simulink model "DAS"  (R2012b)
settings: Solver=FixedStepDiscrete  StartTime=0.0  StopTime=inf  FixedStep=0.1  RelTol=1e-3
PreLoadFcn:
  | if exist('tl_preloadfcn','file'), tl_preloadfcn(gcs,101); end
PostLoadFcn:
  | if exist('tl_postloadfcn','file'), tl_postloadfcn(gcs,101); end
InitFcn:
  | if exist('tlds_init','file'), tlds_init(gcs); end
StartFcn:
  | if exist('tlds_start','file'), tlds_start(gcs); end
StopFcn:
  | if exist('tlds_stop','file'), tlds_stop(gcs); end
undefined symbols (not defined in the file): A, B, C, Dd, DEMO_FAS_Accusti_Threshold_Time, DEMO_FAS_BrakeBooster_Threshold, DEMO_FAS_CC_DELTA, DEMO_FAS_CC_Lvl2_Round, DEMO_FAS_CC_Min_Value, DEMO_FAS_Distance_Treshold_Far, DEMO_FAS_Distance_Treshold_Med, DEMO_FAS_Distance_Treshold_Near, DEMO_FAS_Distronic, DEMO_FAS_Emerg_Brake_Force1, DEMO_FAS_Emerg_Brake_Force2, DEMO_FAS_Emerg_Brake_Time1, DEMO_FAS_Emerg_Brake_Time2, DEMO_FAS_EmergencyBrake, DEMO_FAS_FollowToStop, DEMO_FAS_Limiter, DEMO_FAS_Limiter_DELTA, DEMO_FAS_Neg_Max_ms, DEMO_FAS_Opti_Threshold_Time, DEMO_FAS_Repeater, DEMO_FAS_Repeater_Time, DEMO_FAS_Signdetection, DEMO_FAS_Tempomat
(part 3 of 11)

== system DAS/DEMO_FAS/DEMO_FAS/Subsystem/DEMO_FAS/DEMO_FAS_Funktion/EmergencyBrake ==
  V_Vehicle_ms : Inport
  Distance_Object_m : Inport  Port=2
  V_Obj_rel_ms : Inport  Port=3
  DEMO_FAS_EmergencyBrake : Constant  Description=|  Value=DEMO_FAS_EmergencyBrake  SampleTime=-1  mask(TL_Constant){data={'output',{'variable','DEMO_FAS/p/Components/DEMO_FAS_EmergencyBrake'},'date',735389.66817369207}}
      | Constant block of dSPACE TargetLink.
      | 
      | Output signal keeps the given constant value.
      settings: DeleteFcn=if exist('delete_tlblock','file')==2,delete_tlblock(gcbh);end  NameChangeFcn=if exist('rename_tlblock','file')==2,rename_tlblock(gcbh);end  OpenFcn=if exist('tl_open_blockdlg','file')==2,tl_open_blockdlg(gcbh);else,open_system(gcbh,'parameter');end
      mask Help: eval(['if exist(''tl_online_help'',''file'') == 2, tl_online_help(''Topic'',''TL_Constant''),else, web([''jar:file:///'',matlabroot,''/help/toolbox/simulink/help.jar!/slref/' lower(get_param(gcbh,'Blocktype')) '.html''], ''-helpbrowser''),end'])
      mask Display: plot([-0.05, 1.05, NaN, -0.05, 1.05],[.01, .01, NaN, .99, .99])
  EmergencyBrake_Function : Subsystem
  VERSION_INFO : Subsystem  mask(VERSION_INFO_BLOCK){versinfo_data=struct('modname','DEMO_FAS/DEMO_FAS_Funktion/EmergencyBrake','version','1.1.1','date','29-May-2013','author','YVEDUHR','modtype',3,'variant',0,'remark',{{'~'}},'copyright',['Daimler AG'],'SGMLdescr','','prefix','','pfx_act',0,'ntselect',3,'asize',0), versinfo_string=Model: DEMO_FAS/DEMO_FAS_Funktion/EmergencyBrake\nVersion: 1.1.1\nDate: 29-May-2013\nAuthor: YVEDUHR\nModule: INTERNAL\n\nAll copyrights by Daimler AG}
      mask prompts: versinfo_data "Mask Parameter 1"; versinfo_string "Mask Parameter 2"
      mask help:
      | This is a Version Info Subsystem (empty)
      | All version Information is stored in Parameter "versinfo_data" and displayed
      settings: OpenFcn=edit_subsys_info('init')
      mask Display: disp(versinfo_string);
  BrakeForce_Emergency_pc : Outport
  Acusti_warn_b : Outport  Port=2  InitialOutput=0
  wires:
  DEMO_FAS_EmergencyBrake/1 -> EmergencyBrake_Function/Enable
  V_Obj_rel_ms/1 -> EmergencyBrake_Function/3(V_Obj_rel_ms)
  V_Vehicle_ms/1 -> EmergencyBrake_Function/1(V_Vehicle_ms)
  Distance_Object_m/1 -> EmergencyBrake_Function/2(Distance_Object_m)
  EmergencyBrake_Function/1(BrakeForce_Emergency_pc) -> BrakeForce_Emergency_pc/1
  EmergencyBrake_Function/2(Acusti_warn_b) -> Acusti_warn_b/1

== system DAS/DEMO_FAS/DEMO_FAS/Subsystem/DEMO_FAS/DEMO_FAS_Funktion/FAS_Input ==
  InputBus : Inport
  Bus Creator : BusCreator  Inputs=15
  Bus Selector : BusSelector  OutputSignals=ParkingBrake_b,BrakeForce_pedal_pc,Accelaration_pedal_pc,CruiseControl_b,Limiter_b,LeverUp_stat,LeverDown_stat,V_Vehicle_kmh,V_Sign_kmh,Sign_b,Distance_stat,V_Obj_rel_kmh,Distance_Object_m
  Constant : Constant  Value=3.6  mask(TL_Constant){data={'date',735377.63076421292}}
      settings: CopyFcn=if exist('tl_reset_reviewflag') == 2, tl_reset_reviewflag(gcbh); end  DeleteFcn=if exist('delete_tlblock','file')==2,delete_tlblock(gcbh);end  NameChangeFcn=if exist('rename_tlblock','file')==2,rename_tlblock(gcbh);end  OpenFcn=if exist('tl_open_blockdlg','file')==2,tl_open_blockdlg(gcbh);else,open_system(gcbh,'parameter');end
      mask Help: eval(['if exist(''tl_online_help'',''file'') == 2, tl_online_help(''Topic'',''TL_Constant''),else, web([''jar:file:///'',matlabroot,''/help/toolbox/simulink/help.jar!/slref/' lower(get_param(gcbh,'Blocktype')) '.html''], ''-helpbrowser''),end'])
      mask Display: plot([-0.05, 1.05, NaN, -0.05, 1.05],[.01, .01, NaN, .99, .99])
  Constant1 : Constant  Value=3.6  mask(TL_Constant){data={'date',735377.63076421292}}
      settings: CopyFcn=if exist('tl_reset_reviewflag') == 2, tl_reset_reviewflag(gcbh); end  DeleteFcn=if exist('delete_tlblock','file')==2,delete_tlblock(gcbh);end  NameChangeFcn=if exist('rename_tlblock','file')==2,rename_tlblock(gcbh);end  OpenFcn=if exist('tl_open_blockdlg','file')==2,tl_open_blockdlg(gcbh);else,open_system(gcbh,'parameter');end
      mask Help: eval(['if exist(''tl_online_help'',''file'') == 2, tl_online_help(''Topic'',''TL_Constant''),else, web([''jar:file:///'',matlabroot,''/help/toolbox/simulink/help.jar!/slref/' lower(get_param(gcbh,'Blocktype')) '.html''], ''-helpbrowser''),end'])
      mask Display: plot([-0.05, 1.05, NaN, -0.05, 1.05],[.01, .01, NaN, .99, .99])
  Div : Product  Description=|  Inputs=*/  RndMeth=Zero  mask(TL_Product){data={'logdata',{'plotchannels',[]},'date',734383.73388777778}}
      | Product block of dSPACE TargetLink.
      | 
      | Output signal is equal to the product of the input signals. The input ports are specified according to conventions for Simulink Product blocks.
      settings: CopyFcn=if exist('tl_reset_reviewflag') == 2, tl_reset_reviewflag(gcbh); end  DeleteFcn=if exist('delete_tlblock','file')==2,delete_tlblock(gcbh);end  NameChangeFcn=if exist('rename_tlblock','file')==2,rename_tlblock(gcbh);end  OpenFcn=if exist('tl_open_blockdlg','file')==2,tl_open_blockdlg(gcbh);else,open_system(gcbh,'parameter');end
      mask Help: eval(['if exist(''tl_online_help'',''file'') == 2, tl_online_help(''Topic'',''TL_Product''),else, web([''jar:file:///'',matlabroot,''/help/toolbox/simulink/help.jar!/slref/' lower(get_param(gcbh,'Blocktype')) '.html''], ''-helpbrowser''),end'])
      mask Display: plot([-0.05, 1.05, NaN, -0.05, 1.05],[.01, .01, NaN, .99, .99])
  Div1 : Product  Description=|  Inputs=*/  RndMeth=Zero  mask(TL_Product){data={'logdata',{'plotchannels',[]},'date',734383.73388777778}}
      | Product block of dSPACE TargetLink.
      | 
      | Output signal is equal to the product of the input signals. The input ports are specified according to conventions for Simulink Product blocks.
      settings: CopyFcn=if exist('tl_reset_reviewflag') == 2, tl_reset_reviewflag(gcbh); end  DeleteFcn=if exist('delete_tlblock','file')==2,delete_tlblock(gcbh);end  NameChangeFcn=if exist('rename_tlblock','file')==2,rename_tlblock(gcbh);end  OpenFcn=if exist('tl_open_blockdlg','file')==2,tl_open_blockdlg(gcbh);else,open_system(gcbh,'parameter');end
      mask Help: eval(['if exist(''tl_online_help'',''file'') == 2, tl_online_help(''Topic'',''TL_Product''),else, web([''jar:file:///'',matlabroot,''/help/toolbox/simulink/help.jar!/slref/' lower(get_param(gcbh,'Blocktype')) '.html''], ''-helpbrowser''),end'])
      mask Display: plot([-0.05, 1.05, NaN, -0.05, 1.05],[.01, .01, NaN, .99, .99])
  VERSION_INFO : Subsystem  mask(VERSION_INFO_BLOCK){versinfo_data=struct('modname','DEMO_FAS/DEMO_FAS_Funktion/FAS_Input','version','1.1.1','date','18-Apr-2013','author','YVEDUHR','modtype',3,'variant',0,'remark',{{'~'}},'copyright',['Daimler AG'],'SGMLdescr','','prefix','','pfx_act',0,'ntselect',3,'asize',0), versinfo_string=Model: DEMO_FAS/DEMO_FAS_Funktion/FAS_Input\nVersion: 1.1.1\nDate: 18-Apr-2013\nAuthor: YVEDUHR\nModule: INTERNAL\n\nAll copyrights by Daimler AG}
      mask prompts: versinfo_data "Mask Parameter 1"; versinfo_string "Mask Parameter 2"
      mask help:
      | This is a Version Info Subsystem (empty)
      | All version Information is stored in Parameter "versinfo_data" and displayed
      settings: OpenFcn=edit_subsys_info('init')
      mask Display: disp(versinfo_string);
  FASBus : Outport
  wires:
  InputBus/1 -> Bus Selector/1
  Bus Creator/1 -> FASBus/1  "FASBus"
  Bus Selector/1 -> Bus Creator/1  "<ParkingBrake_b>"
  Bus Selector/6 -> Bus Creator/6  "<LeverUp_stat>"
  Bus Selector/4 -> Bus Creator/4  "<CruiseControl_b>"
  Bus Selector/3 -> Bus Creator/3  "<Accelaration_pedal_pc>"
  Bus Selector/2 -> Bus Creator/2  "<BrakeForce_pedal_pc>"
  Bus Selector/8 -> Div/1, Bus Creator/8  "<V_Vehicle_kmh>"
  Bus Selector/5 -> Bus Creator/5  "<Limiter_b>"
  Bus Selector/7 -> Bus Creator/7  "<LeverDown_stat>"
  Bus Selector/9 -> Bus Creator/10  "<V_Sign_kmh>"
  Bus Selector/10 -> Bus Creator/11  "<Sign_b>"
  Bus Selector/13 -> Bus Creator/15  "<Distance_Object_m>"
  Bus Selector/11 -> Bus Creator/12  "<Distance_stat>"
  Constant/1 -> Div/2
  Div/1 -> Bus Creator/9  "V_Vehicle_ms"
  Bus Selector/12 -> Div1/1, Bus Creator/13  "<V_Obj_rel_kmh>"
  Constant1/1 -> Div1/2
  Div1/1 -> Bus Creator/14  "V_Obj_rel_ms"

== system DAS/DEMO_FAS/DEMO_FAS/Subsystem/DEMO_FAS/DEMO_FAS_Funktion/FollowToStop ==
  V_Vehicle_kmh : Inport
  V_Obj_rel_kmh : Inport  Port=2
  DEMO_FAS_FollowToStop : Constant  Description=|  Value=DEMO_FAS_FollowToStop  SampleTime=-1  mask(TL_Constant){data={'output',{'variable','DEMO_FAS/p/Components/DEMO_FAS_Distronic'},'date',735388.55883950228}}
      | Constant block of dSPACE TargetLink.
      | 
      | Output signal keeps the given constant value.
      settings: DeleteFcn=if exist('delete_tlblock','file')==2,delete_tlblock(gcbh);end  NameChangeFcn=if exist('rename_tlblock','file')==2,rename_tlblock(gcbh);end  OpenFcn=if exist('tl_open_blockdlg','file')==2,tl_open_blockdlg(gcbh);else,open_system(gcbh,'parameter');end
      mask Help: eval(['if exist(''tl_online_help'',''file'') == 2, tl_online_help(''Topic'',''TL_Constant''),else, web([''jar:file:///'',matlabroot,''/help/toolbox/simulink/help.jar!/slref/' lower(get_param(gcbh,'Blocktype')) '.html''], ''-helpbrowser''),end'])
      mask Display: plot([-0.05, 1.05, NaN, -0.05, 1.05],[.01, .01, NaN, .99, .99])
  FollowToStop_Function : Subsystem
  VERSION_INFO : Subsystem  mask(VERSION_INFO_BLOCK){versinfo_data=struct('modname','DEMO_FAS/DEMO_FAS_Funktion/FollowToStop','version','1.1.1','date','28-May-2013','author','YVEDUHR','modtype',3,'variant',0,'remark',{{'~'}},'copyright',['Daimler AG'],'SGMLdescr','','prefix','','pfx_act',0,'ntselect',3,'asize',0), versinfo_string=Model: DEMO_FAS/DEMO_FAS_Funktion/FollowToStop\nVersion: 1.1.1\nDate: 28-May-2013\nAuthor: YVEDUHR\nModule: INTERNAL\n\nAll copyrights by Daimler AG}
      mask prompts: versinfo_data "Mask Parameter 1"; versinfo_string "Mask Parameter 2"
      mask help:
      | This is a Version Info Subsystem (empty)
      | All version Information is stored in Parameter "versinfo_data" and displayed
      settings: OpenFcn=edit_subsys_info('init')
      mask Display: disp(versinfo_string);
  FTS_active_b : Outport
  FTS_Abstand_soll_m : Outport  Port=2
  wires:
  V_Vehicle_kmh/1 -> FollowToStop_Function/1(V_Vehicle_kmh)
  V_Obj_rel_kmh/1 -> FollowToStop_Function/2(V_Obj_rel_kmh)
  DEMO_FAS_FollowToStop/1 -> FollowToStop_Function/Enable
  FollowToStop_Function/1(FTS_active_b) -> FTS_active_b/1
  FollowToStop_Function/2(FTS_Abstand_soll_m) -> FTS_Abstand_soll_m/1

== system DAS/DEMO_FAS/DEMO_FAS/Subsystem/DEMO_FAS/DEMO_FAS_Funktion/Limiter ==
  Limiter_b : Inport
  Accelaration_pedal_pc : Inport  Port=2
  V_Vehicle_kmh : Inport  Port=3
  LeverUp_stat : Inport  Port=4
  LeverDown_stat : Inport  Port=5
  V_Sign_kmh : Inport  Port=6
  Sign_b : Inport  Port=7
  DEMO_FAS_Limiter : Constant  Description=|  Value=DEMO_FAS_Limiter  SampleTime=-1  mask(TL_Constant){data={'output',{'variable','DEMO_FAS/p/Components/DEMO_FAS_Limiter'},'date',735342.475759294}}
      | Constant block of dSPACE TargetLink.
      | 
      | Output signal keeps the given constant value.
      settings: DeleteFcn=if exist('delete_tlblock','file')==2,delete_tlblock(gcbh);end  NameChangeFcn=if exist('rename_tlblock','file')==2,rename_tlblock(gcbh);end  OpenFcn=if exist('tl_open_blockdlg','file')==2,tl_open_blockdlg(gcbh);else,open_system(gcbh,'parameter');end
      mask Help: eval(['if exist(''tl_online_help'',''file'') == 2, tl_online_help(''Topic'',''TL_Constant''),else, web([''jar:file:///'',matlabroot,''/help/toolbox/simulink/help.jar!/slref/' lower(get_param(gcbh,'Blocktype')) '.html''], ''-helpbrowser''),end'])
      mask Display: plot([-0.05, 1.05, NaN, -0.05, 1.05],[.01, .01, NaN, .99, .99])
  Limiter_Function : Subsystem
  VERSION_INFO : Subsystem  mask(VERSION_INFO_BLOCK){versinfo_data=struct('modname','DEMO_FAS/DEMO_FAS_Funktion/Limiter','version','1.1.1','date','18-Apr-2013','author','YVEDUHR','modtype',3,'variant',0,'remark',{{['~15-05-2013: Sign Detection added']}},'copyright',['Daimler AG'],'SGMLdescr','','prefix','','pfx_act',0,'ntselect',3,'asize',0), versinfo_string=Model: DEMO_FAS/DEMO_FAS_Funktion/Limiter\nVersion: 1.1.1\nDate: 18-Apr-2013\nAuthor: YVEDUHR\nModule: INTERNAL\n\nAll copyrights by Daimler AG}
      mask prompts: versinfo_data "Mask Parameter 1"; versinfo_string "Mask Parameter 2"
      mask help:
      | This is a Version Info Subsystem (empty)
      | All version Information is stored in Parameter "versinfo_data" and displayed
      settings: OpenFcn=edit_subsys_info('init')
      mask Display: disp(versinfo_string);
  VMax_kmh : Outport
  Limiter_active_b : Outport  Port=2  InitialOutput=0
  wires:
  Limiter_b/1 -> Limiter_Function/1(Limiter_b)
  Accelaration_pedal_pc/1 -> Limiter_Function/2(Accelaration_pedal_pc)
  V_Vehicle_kmh/1 -> Limiter_Function/3(V_Vehicle_kmh)
  LeverUp_stat/1 -> Limiter_Function/4(LeverUp_stat)
  LeverDown_stat/1 -> Limiter_Function/5(LeverDown_stat)
  V_Sign_kmh/1 -> Limiter_Function/6(V_Sign_kmh)
  Sign_b/1 -> Limiter_Function/7(Sign_b)
  Limiter_Function/1(VMax_kmh) -> VMax_kmh/1
  Limiter_Function/2(Limiter_active_b) -> Limiter_active_b/1
  DEMO_FAS_Limiter/1 -> Limiter_Function/Enable

== system DAS/DEMO_FAS/DEMO_FAS/Subsystem/DEMO_FAS/DEMO_FAS_Funktion/Tempomat ==
  ParkingBrake_b : Inport
  BrakeForce_pedal_pc : Inport  Port=2
  CruiseControl_b : Inport  Port=3
  V_Vehicle_kmh : Inport  Port=4
  Limiter_b : Inport  Port=5
  LeverUp_Stat : Inport  Port=6
  LeverDown_Stat : Inport  Port=7
  FTS_active_b : Inport  Port=8
  DEMO_FAS_Tempomat : Constant  Description=|  Value=DEMO_FAS_Tempomat  SampleTime=-1  mask(TL_Constant){data={'output',{'variable','DEMO_FAS/p/Components/DEMO_FAS_Tempomat'},'date',735441.60748548608}}
      | Constant block of dSPACE TargetLink.
      | 
      | Output signal keeps the given constant value.
      settings: DeleteFcn=if exist('delete_tlblock','file')==2,delete_tlblock(gcbh);end  NameChangeFcn=if exist('rename_tlblock','file')==2,rename_tlblock(gcbh);end  OpenFcn=if exist('tl_open_blockdlg','file')==2,tl_open_blockdlg(gcbh);else,open_system(gcbh,'parameter');end
      mask Help: eval(['if exist(''tl_online_help'',''file'') == 2, tl_online_help(''Topic'',''TL_Constant''),else, web([''jar:file:///'',matlabroot,''/help/toolbox/simulink/help.jar!/slref/' lower(get_param(gcbh,'Blocktype')) '.html''], ''-helpbrowser''),end'])
      mask Display: plot([-0.05, 1.05, NaN, -0.05, 1.05],[.01, .01, NaN, .99, .99])
  Tempomat_Function : Subsystem
  VERSION_INFO : Subsystem  mask(VERSION_INFO_BLOCK){versinfo_data=struct('modname','DEMO_FAS/DEMO_FAS_Funktion/Tempomat','version','1.1.1','date','18-Apr-2013','author','YVEDUHR','modtype',3,'variant',0,'remark',{{'~'}},'copyright',['Daimler AG'],'SGMLdescr','','prefix','','pfx_act',0,'ntselect',3,'asize',0), versinfo_string=Model: DEMO_FAS/DEMO_FAS_Funktion/Tempomat\nVersion: 1.1.1\nDate: 18-Apr-2013\nAuthor: YVEDUHR\nModule: INTERNAL\n\nAll copyrights by Daimler AG}
      mask prompts: versinfo_data "Mask Parameter 1"; versinfo_string "Mask Parameter 2"
      mask help:
      | This is a Version Info Subsystem (empty)
      | All version Information is stored in Parameter "versinfo_data" and displayed
      settings: OpenFcn=edit_subsys_info('init')
      mask Display: disp(versinfo_string);
  V_CC_delta_kmh : Outport
  CC_active_b : Outport  Port=2  InitialOutput=0
  wires:
  ParkingBrake_b/1 -> Tempomat_Function/1(ParkingBrake_b)
  BrakeForce_pedal_pc/1 -> Tempomat_Function/2(BrakeForce_pedal_pc)
  CruiseControl_b/1 -> Tempomat_Function/3(CruiseControl_b)
  V_Vehicle_kmh/1 -> Tempomat_Function/4(V_Vehicle_kmh)
  Limiter_b/1 -> Tempomat_Function/5(Limiter_b)
  LeverUp_Stat/1 -> Tempomat_Function/6(LeverUp_Stat)
  LeverDown_Stat/1 -> Tempomat_Function/7(LeverDown_Stat)
  FTS_active_b/1 -> Tempomat_Function/8(FTS_active_b)
  Tempomat_Function/1(V_CC_delta_kmh) -> V_CC_delta_kmh/1
  Tempomat_Function/2(CC_active_b) -> CC_active_b/1
  DEMO_FAS_Tempomat/1 -> Tempomat_Function/Enable

== system DAS/DEMO_FAS/DEMO_FAS/Subsystem/DEMO_FAS/DEMO_FAS_Funktion/VERSION_INFO ==
  Copyright : Subsystem
      mask help: Copyright
      mask Display: disp('All copyrights by DaimlerChrysler');

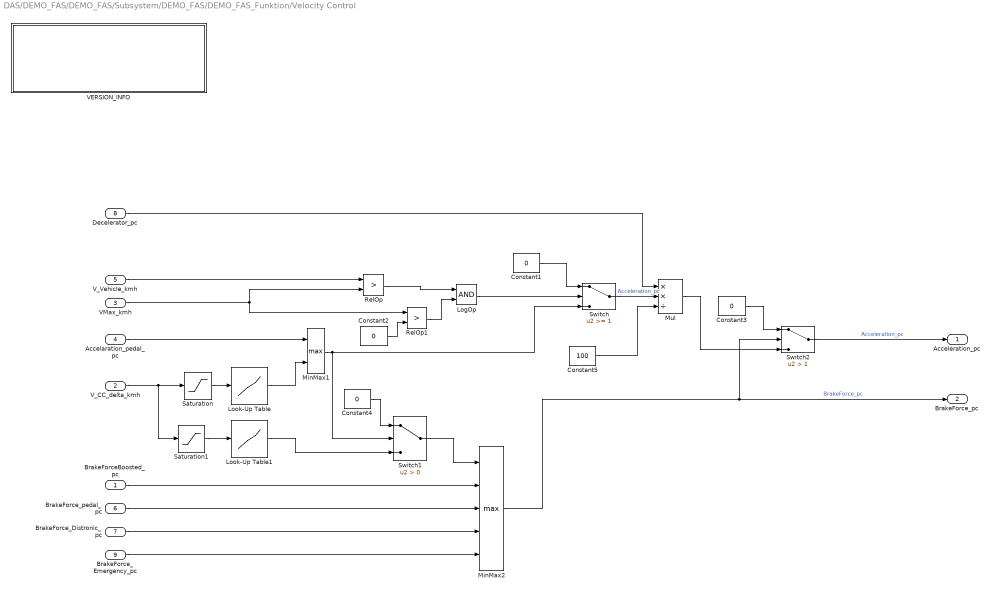
== system DAS/DEMO_FAS/DEMO_FAS/Subsystem/DEMO_FAS/DEMO_FAS_Funktion/Velocity Control ==
  BrakeForceBoosted_pc : Inport
  V_CC_delta_kmh : Inport  Port=2
  VMax_kmh : Inport  Port=3
  Accelaration_pedal_pc : Inport  Port=4
  V_Vehicle_kmh : Inport  Port=5
  BrakeForce_pedal_pc : Inport  Port=6
  BrakeForce_Distronic_pc : Inport  Port=7
  Decelerator_pc : Inport  Port=8
  BrakeForce_Emergency_pc : Inport  Port=9
  Constant{1..4} (4 alike) : Constant  Value=0  mask(TL_Constant){data={'date',735342.59861445602}}
      settings: CopyFcn=if exist('tl_reset_reviewflag') == 2, tl_reset_reviewflag(gcbh); end  DeleteFcn=if exist('delete_tlblock','file')==2,delete_tlblock(gcbh);end  NameChangeFcn=if exist('rename_tlblock','file')==2,rename_tlblock(gcbh);end  OpenFcn=if exist('tl_open_blockdlg','file')==2,tl_open_blockdlg(gcbh);else,open_system(gcbh,'parameter');end
      mask Help: eval(['if exist(''tl_online_help'',''file'') == 2, tl_online_help(''Topic'',''TL_Constant''),else, web([''jar:file:///'',matlabroot,''/help/toolbox/simulink/help.jar!/slref/' lower(get_param(gcbh,'Blocktype')) '.html''], ''-helpbrowser''),end'])
      mask Display: plot([-0.05, 1.05, NaN, -0.05, 1.05],[.01, .01, NaN, .99, .99])
  Constant5 : Constant  Value=100  mask(TL_Constant){data={'date',735389.67880475696}}
      settings: CopyFcn=if exist('tl_reset_reviewflag') == 2, tl_reset_reviewflag(gcbh); end  DeleteFcn=if exist('delete_tlblock','file')==2,delete_tlblock(gcbh);end  NameChangeFcn=if exist('rename_tlblock','file')==2,rename_tlblock(gcbh);end  OpenFcn=if exist('tl_open_blockdlg','file')==2,tl_open_blockdlg(gcbh);else,open_system(gcbh,'parameter');end
      mask Help: eval(['if exist(''tl_online_help'',''file'') == 2, tl_online_help(''Topic'',''TL_Constant''),else, web([''jar:file:///'',matlabroot,''/help/toolbox/simulink/help.jar!/slref/' lower(get_param(gcbh,'Blocktype')) '.html''], ''-helpbrowser''),end'])
      mask Display: plot([-0.05, 1.05, NaN, -0.05, 1.05],[.01, .01, NaN, .99, .99])
  LogOp : Logic  Description=|  AllPortsSameDT=off  mask(TL_LogicalOperator){data={'logdata',{'plotchannels',[]},'date',734383.73388633097}}
      | Logical operator block of dSPACE TargetLink.
      | 
      | The Logical Operator block performs any of these logical operations on its inputs: AND, OR, NAND, NOR, XOR, and NOT. A nonzero input is treated as TRUE (1), a zero input as FALSE (0). The output depends on the selected operator. The output is 1 if TRUE and 0 if FALSE.
      settings: DeleteFcn=if exist('delete_tlblock','file')==2,delete_tlblock(gcbh);end  NameChangeFcn=if exist('rename_tlblock','file')==2,rename_tlblock(gcbh);end  OpenFcn=if exist('tl_open_blockdlg','file')==2,tl_open_blockdlg(gcbh);else,open_system(gcbh,'parameter');end
      mask Help: eval(['if exist(''tl_online_help'',''file'') == 2, tl_online_help(''Topic'',''TL_LogicalOperator''),else, web([''jar:file:///'',matlabroot,''/help/toolbox/simulink/help.jar!/slref/' lower(get_param(gcbh,'Blocktype')) '.html''], ''-helpbrowser''),end'])
      mask Display: plot([-0.05, 1.05, NaN, -0.05, 1.05],[.01, .01, NaN, .99, .99])
  Look-Up Table : Lookup_n-D  NumberOfTableDimensions=1  BreakpointsForDimension1=[0 1 5 10]  BreakpointsForDimension2=[1:3]  IndexSearchMethod=Linear search  Table=[0 20 60 100]  ExtrapMethod=Clip  RndMeth=Simplest  InputSameDT=on  mask(TL_Lookup1D){data={'input',{'type','Int16'},'table',{'type','Int16'},'date',735342.59760248847}}
      settings: CopyFcn=if exist('tl_reset_reviewflag') == 2, tl_reset_reviewflag(gcbh); end  DeleteFcn=if exist('delete_tlblock','file')==2,delete_tlblock(gcbh);end  NameChangeFcn=if exist('rename_tlblock','file')==2,rename_tlblock(gcbh);end  OpenFcn=if exist('tl_open_blockdlg','file')==2,tl_open_blockdlg(gcbh);else,open_system(gcbh,'parameter');end
      mask Help: eval(['if exist(''tl_online_help'',''file'') == 2, tl_online_help(''Topic'',''TL_Lookup1D''),else, web([''jar:file:///'',matlabroot,''/help/toolbox/simulink/help.jar!/slref/' lower(get_param(gcbh,'Blocktype')) '.html''], ''-helpbrowser''),end'])
      mask Display: plot([-0.05, 1.05, NaN, -0.05, 1.05],[.01, .01, NaN, .99, .99])
  Look-Up Table1 : Lookup_n-D  NumberOfTableDimensions=1  BreakpointsForDimension1=[-10 -5 -1 0]  BreakpointsForDimension2=[1:3]  IndexSearchMethod=Linear search  Table=[100 40 5 0]  ExtrapMethod=Clip  RndMeth=Simplest  InputSameDT=on  mask(TL_Lookup1D){data={'input',{'type','Int16'},'table',{'type','Int16'},'date',735350.38531726855}}
      settings: CopyFcn=if exist('tl_reset_reviewflag') == 2, tl_reset_reviewflag(gcbh); end  DeleteFcn=if exist('delete_tlblock','file')==2,delete_tlblock(gcbh);end  NameChangeFcn=if exist('rename_tlblock','file')==2,rename_tlblock(gcbh);end  OpenFcn=if exist('tl_open_blockdlg','file')==2,tl_open_blockdlg(gcbh);else,open_system(gcbh,'parameter');end
      mask Help: eval(['if exist(''tl_online_help'',''file'') == 2, tl_online_help(''Topic'',''TL_Lookup1D''),else, web([''jar:file:///'',matlabroot,''/help/toolbox/simulink/help.jar!/slref/' lower(get_param(gcbh,'Blocktype')) '.html''], ''-helpbrowser''),end'])
      mask Display: plot([-0.05, 1.05, NaN, -0.05, 1.05],[.01, .01, NaN, .99, .99])
  MinMax1 : MinMax  Description=|  Function=max  Inputs=2  mask(TL_MinMax){data={'logdata',{'plotchannels',[]},'date',735342.59806893521}}
      | MinMax block of dSPACE TargetLink.
      | 
      | The MinMax block outputs either the minimum or the maximum element or elements of the input(s). If the block has one input port, the block outputs a scalar that is the minimum or maximum element of the input vector. If the block has more than one input port, the block performs an element-by-element comparison of the input vectors. Each element of the block output vector is the result of the comparison of the elements of the input vectors. The output of this block is equal to the greater or smaller input depending on the selected function.
      settings: CopyFcn=if exist('tl_reset_reviewflag') == 2, tl_reset_reviewflag(gcbh); end  DeleteFcn=if exist('delete_tlblock','file')==2,delete_tlblock(gcbh);end  NameChangeFcn=if exist('rename_tlblock','file')==2,rename_tlblock(gcbh);end  OpenFcn=if exist('tl_open_blockdlg','file')==2,tl_open_blockdlg(gcbh);else,open_system(gcbh,'parameter');end
      mask Help: eval(['if exist(''tl_online_help'',''file'') == 2, tl_online_help(''Topic'',''TL_MinMax''),else, web([''jar:file:///'',matlabroot,''/help/toolbox/simulink/help.jar!/slref/' lower(get_param(gcbh,'Blocktype')) '.html''], ''-helpbrowser''),end'])
      mask Display: plot([-0.05, 1.05, NaN, -0.05, 1.05],[.01, .01, NaN, .99, .99])
  MinMax2 : MinMax  Description=|  Function=max  Inputs=5  mask(TL_MinMax){data={'logdata',{'plotchannels',[]},'date',735383.5334921875}}
      | MinMax block of dSPACE TargetLink.
      | 
      | The MinMax block outputs either the minimum or the maximum element or elements of the input(s). If the block has one input port, the block outputs a scalar that is the minimum or maximum element of the input vector. If the block has more than one input port, the block performs an element-by-element comparison of the input vectors. Each element of the block output vector is the result of the comparison of the elements of the input vectors. The output of this block is equal to the greater or smaller input depending on the selected function.
      settings: CopyFcn=if exist('tl_reset_reviewflag') == 2, tl_reset_reviewflag(gcbh); end  DeleteFcn=if exist('delete_tlblock','file')==2,delete_tlblock(gcbh);end  NameChangeFcn=if exist('rename_tlblock','file')==2,rename_tlblock(gcbh);end  OpenFcn=if exist('tl_open_blockdlg','file')==2,tl_open_blockdlg(gcbh);else,open_system(gcbh,'parameter');end
      mask Help: eval(['if exist(''tl_online_help'',''file'') == 2, tl_online_help(''Topic'',''TL_MinMax''),else, web([''jar:file:///'',matlabroot,''/help/toolbox/simulink/help.jar!/slref/' lower(get_param(gcbh,'Blocktype')) '.html''], ''-helpbrowser''),end'])
      mask Display: plot([-0.05, 1.05, NaN, -0.05, 1.05],[.01, .01, NaN, .99, .99])
  Mul : Product  Description=|  Inputs=**/  RndMeth=Zero  mask(TL_Product){data={'logdata',{'plotchannels',[]},'date',735389.67847318284}}
      | Product block of dSPACE TargetLink.
      | 
      | Output signal is equal to the product of the input signals. The input ports are specified according to conventions for Simulink Product blocks.
      settings: CopyFcn=if exist('tl_reset_reviewflag') == 2, tl_reset_reviewflag(gcbh); end  DeleteFcn=if exist('delete_tlblock','file')==2,delete_tlblock(gcbh);end  NameChangeFcn=if exist('rename_tlblock','file')==2,rename_tlblock(gcbh);end  OpenFcn=if exist('tl_open_blockdlg','file')==2,tl_open_blockdlg(gcbh);else,open_system(gcbh,'parameter');end
      mask Help: eval(['if exist(''tl_online_help'',''file'') == 2, tl_online_help(''Topic'',''TL_Product''),else, web([''jar:file:///'',matlabroot,''/help/toolbox/simulink/help.jar!/slref/' lower(get_param(gcbh,'Blocktype')) '.html''], ''-helpbrowser''),end'])
      mask Display: plot([-0.05, 1.05, NaN, -0.05, 1.05],[.01, .01, NaN, .99, .99])
  RelOp : RelationalOperator  Description=|  Operator=>  mask(TL_RelationalOperator){data={'logdata',{'plotchannels',[]},'date',735342.59901829856}}
      | Relational operator block of dSPACE TargetLink.
      | 
      | This block performs a relational operation on its two inputs u1 and u2 and produces output according to the following table.
      | If the result is TRUE, the output is 1; if FALSE, it is 0.
      | 
      | Operator   Output
      |  ==        TRUE if u1 is equal to u2
      |  !=        TRUE if u1 is not equal to u2
      |  <         TRUE if u1 is less than u2
      |  <=        TRUE if u1 is less than or equal to u2
      |  >=        TRUE if u1 is greater than or equal to u2
      |  >         TRUE if u1 is greater than u2
      settings: DeleteFcn=if exist('delete_tlblock','file')==2,delete_tlblock(gcbh);end  NameChangeFcn=if exist('rename_tlblock','file')==2,rename_tlblock(gcbh);end  OpenFcn=if exist('tl_open_blockdlg','file')==2,tl_open_blockdlg(gcbh);else,open_system(gcbh,'parameter');end
      mask Help: eval(['if exist(''tl_online_help'',''file'') == 2, tl_online_help(''Topic'',''TL_RelationalOperator''),else, web([''jar:file:///'',matlabroot,''/help/toolbox/simulink/help.jar!/slref/' lower(get_param(gcbh,'Blocktype')) '.html''], ''-helpbrowser''),end'])
      mask Display: plot([-0.05, 1.05, NaN, -0.05, 1.05],[.01, .01, NaN, .99, .99])
  RelOp1 : RelationalOperator  Description=|  Operator=>  mask(TL_RelationalOperator){data={'logdata',{'plotchannels',[]},'date',735342.59901829856}}
      | Relational operator block of dSPACE TargetLink.
      | 
      | This block performs a relational operation on its two inputs u1 and u2 and produces output according to the following table.
      | If the result is TRUE, the output is 1; if FALSE, it is 0.
      | 
      | Operator   Output
      |  ==        TRUE if u1 is equal to u2
      |  !=        TRUE if u1 is not equal to u2
      |  <         TRUE if u1 is less than u2
      |  <=        TRUE if u1 is less than or equal to u2
      |  >=        TRUE if u1 is greater than or equal to u2
      |  >         TRUE if u1 is greater than u2
      settings: DeleteFcn=if exist('delete_tlblock','file')==2,delete_tlblock(gcbh);end  NameChangeFcn=if exist('rename_tlblock','file')==2,rename_tlblock(gcbh);end  OpenFcn=if exist('tl_open_blockdlg','file')==2,tl_open_blockdlg(gcbh);else,open_system(gcbh,'parameter');end
      mask Help: eval(['if exist(''tl_online_help'',''file'') == 2, tl_online_help(''Topic'',''TL_RelationalOperator''),else, web([''jar:file:///'',matlabroot,''/help/toolbox/simulink/help.jar!/slref/' lower(get_param(gcbh,'Blocktype')) '.html''], ''-helpbrowser''),end'])
      mask Display: plot([-0.05, 1.05, NaN, -0.05, 1.05],[.01, .01, NaN, .99, .99])
  Saturation : Saturate  UpperLimit=10  LowerLimit=0  mask(TL_Saturate){data={'date',735342.62833549769}}
      settings: CopyFcn=if exist('tl_reset_reviewflag') == 2, tl_reset_reviewflag(gcbh); end  DeleteFcn=if exist('delete_tlblock','file')==2,delete_tlblock(gcbh);end  NameChangeFcn=if exist('rename_tlblock','file')==2,rename_tlblock(gcbh);end  OpenFcn=if exist('tl_open_blockdlg','file')==2,tl_open_blockdlg(gcbh);else,open_system(gcbh,'parameter');end
      mask Help: eval(['if exist(''tl_online_help'',''file'') == 2, tl_online_help(''Topic'',''TL_Saturate''),else, web([''jar:file:///'',matlabroot,''/help/toolbox/simulink/help.jar!/slref/' lower(get_param(gcbh,'Blocktype')) '.html''], ''-helpbrowser''),end'])
      mask Display: plot([-0.05, 1.05, NaN, -0.05, 1.05],[.01, .01, NaN, .99, .99])
  Saturation1 : Saturate  UpperLimit=0  LowerLimit=-10  mask(TL_Saturate){data={'date',735350.38457865745}}
      settings: CopyFcn=if exist('tl_reset_reviewflag') == 2, tl_reset_reviewflag(gcbh); end  DeleteFcn=if exist('delete_tlblock','file')==2,delete_tlblock(gcbh);end  NameChangeFcn=if exist('rename_tlblock','file')==2,rename_tlblock(gcbh);end  OpenFcn=if exist('tl_open_blockdlg','file')==2,tl_open_blockdlg(gcbh);else,open_system(gcbh,'parameter');end
      mask Help: eval(['if exist(''tl_online_help'',''file'') == 2, tl_online_help(''Topic'',''TL_Saturate''),else, web([''jar:file:///'',matlabroot,''/help/toolbox/simulink/help.jar!/slref/' lower(get_param(gcbh,'Blocktype')) '.html''], ''-helpbrowser''),end'])
      mask Display: plot([-0.05, 1.05, NaN, -0.05, 1.05],[.01, .01, NaN, .99, .99])
  Switch : Switch  Threshold=1  mask(TL_Switch){data={'date',735342.59663996531}}
      settings: CopyFcn=if exist('tl_reset_reviewflag') == 2, tl_reset_reviewflag(gcbh); end  DeleteFcn=if exist('delete_tlblock','file')==2,delete_tlblock(gcbh);end  NameChangeFcn=if exist('rename_tlblock','file')==2,rename_tlblock(gcbh);end  OpenFcn=if exist('tl_open_blockdlg','file')==2,tl_open_blockdlg(gcbh);else,open_system(gcbh,'parameter');end
      mask Help: eval(['if exist(''tl_online_help'',''file'') == 2, tl_online_help(''Topic'',''TL_Switch''),else, web([''jar:file:///'',matlabroot,''/help/toolbox/simulink/help.jar!/slref/' lower(get_param(gcbh,'Blocktype')) '.html''], ''-helpbrowser''),end'])
      mask Display: plot([-0.05, 1.05, NaN, -0.05, 1.05],[.01, .01, NaN, .99, .99])
  Switch1 : Switch  Criteria=u2 > Threshold  mask(TL_Switch){data={'date',735350.47172620369}}
      settings: CopyFcn=if exist('tl_reset_reviewflag') == 2, tl_reset_reviewflag(gcbh); end  DeleteFcn=if exist('delete_tlblock','file')==2,delete_tlblock(gcbh);end  NameChangeFcn=if exist('rename_tlblock','file')==2,rename_tlblock(gcbh);end  OpenFcn=if exist('tl_open_blockdlg','file')==2,tl_open_blockdlg(gcbh);else,open_system(gcbh,'parameter');end
      mask Help: eval(['if exist(''tl_online_help'',''file'') == 2, tl_online_help(''Topic'',''TL_Switch''),else, web([''jar:file:///'',matlabroot,''/help/toolbox/simulink/help.jar!/slref/' lower(get_param(gcbh,'Blocktype')) '.html''], ''-helpbrowser''),end'])
      mask Display: plot([-0.05, 1.05, NaN, -0.05, 1.05],[.01, .01, NaN, .99, .99])
  Switch2 : Switch  Criteria=u2 > Threshold  Threshold=1  mask(TL_Switch){data={'date',735389.69151828706}}
      settings: CopyFcn=if exist('tl_reset_reviewflag') == 2, tl_reset_reviewflag(gcbh); end  DeleteFcn=if exist('delete_tlblock','file')==2,delete_tlblock(gcbh);end  NameChangeFcn=if exist('rename_tlblock','file')==2,rename_tlblock(gcbh);end  OpenFcn=if exist('tl_open_blockdlg','file')==2,tl_open_blockdlg(gcbh);else,open_system(gcbh,'parameter');end
      mask Help: eval(['if exist(''tl_online_help'',''file'') == 2, tl_online_help(''Topic'',''TL_Switch''),else, web([''jar:file:///'',matlabroot,''/help/toolbox/simulink/help.jar!/slref/' lower(get_param(gcbh,'Blocktype')) '.html''], ''-helpbrowser''),end'])
      mask Display: plot([-0.05, 1.05, NaN, -0.05, 1.05],[.01, .01, NaN, .99, .99])
  VERSION_INFO : Subsystem  mask(VERSION_INFO_BLOCK){versinfo_data=struct('modname',['DEMO_FAS/DEMO_FAS_Funktion/Velocity Control'],'version','1.1.1','date','18-Apr-2013','author','YVEDUHR','modtype',3,'variant',0,'remark',{{'~'}},'copyright',['Daimler AG'],'SGMLdescr','','prefix','','pfx_act',0,'ntselect',3,'asize',0), versinfo_string=Model: DEMO_FAS/DEMO_FAS_Funktion/Velocity Control\nVersion: 1.1.1\nDate: 18-Apr-2013\nAuthor: YVEDUHR\nModule: INTERNAL\n\nAll copyrights by Daimler AG}
      mask prompts: versinfo_data "Mask Parameter 1"; versinfo_string "Mask Parameter 2"
      mask help:
      | This is a Version Info Subsystem (empty)
      | All version Information is stored in Parameter "versinfo_data" and displayed
      settings: OpenFcn=edit_subsys_info('init')
      mask Display: disp(versinfo_string);
  Acceleration_pc : Outport
  BrakeForce_pc : Outport  Port=2
  wires:
  Constant1/1 -> Switch/1
  RelOp1/1 -> LogOp/2
  RelOp/1 -> LogOp/1
  LogOp/1 -> Switch/2
  V_CC_delta_kmh/1 -> Saturation1/1, Saturation/1
  Look-Up Table/1 -> MinMax1/2
  V_Vehicle_kmh/1 -> RelOp/1
  VMax_kmh/1 -> RelOp1/1, RelOp/2
  Accelaration_pedal_pc/1 -> MinMax1/1
  Switch2/1 -> Acceleration_pc/1  "Acceleration_pc"
  Constant2/1 -> RelOp1/2
  Saturation/1 -> Look-Up Table/1
  Saturation1/1 -> Look-Up Table1/1
  BrakeForceBoosted_pc/1 -> MinMax2/2
  Look-Up Table1/1 -> Switch1/3
  BrakeForce_pedal_pc/1 -> MinMax2/3
  MinMax2/1 -> Switch2/2, BrakeForce_pc/1  "BrakeForce_pc"
  Switch1/1 -> MinMax2/1
  MinMax1/1 -> Switch1/2, Switch/3
  Constant4/1 -> Switch1/1
  BrakeForce_Emergency_pc/1 -> MinMax2/5
  BrakeForce_Distronic_pc/1 -> MinMax2/4
  Switch/1 -> Mul/2  "Acceleration_pc"
  Constant3/1 -> Switch2/1
  Decelerator_pc/1 -> Mul/1
  Mul/1 -> Switch2/3
  Constant5/1 -> Mul/3

== system DAS/DEMO_FAS/DEMO_FAS/Subsystem/DEMO_FAS/DEMO_FAS_Funktion/BrakeAssistant/Brake_Booster ==
  BrakeForce_pedal_pc : Inport
  Constant : Constant  Value=100  mask(TL_Constant){data={'date',735349.62176872685}}
      settings: CopyFcn=if exist('tl_reset_reviewflag') == 2, tl_reset_reviewflag(gcbh); end  DeleteFcn=if exist('delete_tlblock','file')==2,delete_tlblock(gcbh);end  NameChangeFcn=if exist('rename_tlblock','file')==2,rename_tlblock(gcbh);end  OpenFcn=if exist('tl_open_blockdlg','file')==2,tl_open_blockdlg(gcbh);else,open_system(gcbh,'parameter');end
      mask Help: eval(['if exist(''tl_online_help'',''file'') == 2, tl_online_help(''Topic'',''TL_Constant''),else, web([''jar:file:///'',matlabroot,''/help/toolbox/simulink/help.jar!/slref/' lower(get_param(gcbh,'Blocktype')) '.html''], ''-helpbrowser''),end'])
      mask Display: plot([-0.05, 1.05, NaN, -0.05, 1.05],[.01, .01, NaN, .99, .99])
  DEMO_FAS_BrakeBooster_Threshold : Constant  Description=|  Value=DEMO_FAS_BrakeBooster_Threshold  SampleTime=-1  mask(TL_Constant){data={'output',{'variable','DEMO_FAS/p/Components/DEMO_FAS_BrakeBooster_Threshold'},'date',735354.40793805558}}
      | Constant block of dSPACE TargetLink.
      | 
      | Output signal keeps the given constant value.
      settings: DeleteFcn=if exist('delete_tlblock','file')==2,delete_tlblock(gcbh);end  NameChangeFcn=if exist('rename_tlblock','file')==2,rename_tlblock(gcbh);end  OpenFcn=if exist('tl_open_blockdlg','file')==2,tl_open_blockdlg(gcbh);else,open_system(gcbh,'parameter');end
      mask Help: eval(['if exist(''tl_online_help'',''file'') == 2, tl_online_help(''Topic'',''TL_Constant''),else, web([''jar:file:///'',matlabroot,''/help/toolbox/simulink/help.jar!/slref/' lower(get_param(gcbh,'Blocktype')) '.html''], ''-helpbrowser''),end'])
      mask Display: plot([-0.05, 1.05, NaN, -0.05, 1.05],[.01, .01, NaN, .99, .99])
  RelOp : RelationalOperator  Description=|  mask(TL_RelationalOperator){data={'logdata',{'plotchannels',[]},'date',735349.6188950463}}
      | Relational operator block of dSPACE TargetLink.
      | 
      | This block performs a relational operation on its two inputs u1 and u2 and produces output according to the following table.
      | If the result is TRUE, the output is 1; if FALSE, it is 0.
      | 
      | Operator   Output
      |  ==        TRUE if u1 is equal to u2
      |  !=        TRUE if u1 is not equal to u2
      |  <         TRUE if u1 is less than u2
      |  <=        TRUE if u1 is less than or equal to u2
      |  >=        TRUE if u1 is greater than or equal to u2
      |  >         TRUE if u1 is greater than u2
      settings: DeleteFcn=if exist('delete_tlblock','file')==2,delete_tlblock(gcbh);end  NameChangeFcn=if exist('rename_tlblock','file')==2,rename_tlblock(gcbh);end  OpenFcn=if exist('tl_open_blockdlg','file')==2,tl_open_blockdlg(gcbh);else,open_system(gcbh,'parameter');end
      mask Help: eval(['if exist(''tl_online_help'',''file'') == 2, tl_online_help(''Topic'',''TL_RelationalOperator''),else, web([''jar:file:///'',matlabroot,''/help/toolbox/simulink/help.jar!/slref/' lower(get_param(gcbh,'Blocktype')) '.html''], ''-helpbrowser''),end'])
      mask Display: plot([-0.05, 1.05, NaN, -0.05, 1.05],[.01, .01, NaN, .99, .99])
  Switch : Switch  Threshold=1  mask(TL_Switch){data={'date',735349.62130812497}}
      settings: CopyFcn=if exist('tl_reset_reviewflag') == 2, tl_reset_reviewflag(gcbh); end  DeleteFcn=if exist('delete_tlblock','file')==2,delete_tlblock(gcbh);end  NameChangeFcn=if exist('rename_tlblock','file')==2,rename_tlblock(gcbh);end  OpenFcn=if exist('tl_open_blockdlg','file')==2,tl_open_blockdlg(gcbh);else,open_system(gcbh,'parameter');end
      mask Help: eval(['if exist(''tl_online_help'',''file'') == 2, tl_online_help(''Topic'',''TL_Switch''),else, web([''jar:file:///'',matlabroot,''/help/toolbox/simulink/help.jar!/slref/' lower(get_param(gcbh,'Blocktype')) '.html''], ''-helpbrowser''),end'])
      mask Display: plot([-0.05, 1.05, NaN, -0.05, 1.05],[.01, .01, NaN, .99, .99])
  VERSION_INFO : Subsystem  mask(VERSION_INFO_BLOCK){versinfo_data=struct('modname','DEMO_FAS/DEMO_FAS_Funktion/BrakeAssistant/Brake_Booster','version','1.1.1','date','26-Apr-2013','author','YVEDUHR','modtype',3,'variant',0,'remark',{{'~'}},'copyright',['Daimler AG'],'SGMLdescr','','prefix','','pfx_act',0,'ntselect',3,'asize',0), versinfo_string=Model: DEMO_FAS/DEMO_FAS_Funktion/BrakeAssistant/Brake_Booster\nVersion: 1.1.1\nDate: 26-Apr-2013\nAuthor: YVEDUHR\nModule: INTERNAL\n\nAll copyrights by Daimler AG}
      mask prompts: versinfo_data "Mask Parameter 1"; versinfo_string "Mask Parameter 2"
      mask help:
      | This is a Version Info Subsystem (empty)
      | All version Information is stored in Parameter "versinfo_data" and displayed
      settings: OpenFcn=edit_subsys_info('init')
      mask Display: disp(versinfo_string);
  BrakeForceBoosted_pc : Outport  OutputWhenDisabled=reset  InitialOutput=0
  wires:
  BrakeForce_pedal_pc/1 -> Switch/3, RelOp/1
  RelOp/1 -> Switch/2
  DEMO_FAS_BrakeBooster_Threshold/1 -> RelOp/2
  Constant/1 -> Switch/1
  Switch/1 -> BrakeForceBoosted_pc/1  "BrakeForceBoosted_pc"

== system DAS/DEMO_FAS/DEMO_FAS/Subsystem/DEMO_FAS/DEMO_FAS_Funktion/BrakeAssistant/VERSION_INFO ==
  Copyright : Subsystem
      mask help: Copyright
      mask Display: disp('All copyrights by DaimlerChrysler');

== system DAS/DEMO_FAS/DEMO_FAS/Subsystem/DEMO_FAS/DEMO_FAS_Funktion/Distancewarner/Distancewarner_Function ==
  V_Vehicle_ms : Inport
  Distance_Object_m : Inport  Port=2
  DEMO_FAS_Accusti_Threshold_Time : Constant  Description=|  Value=DEMO_FAS_Accusti_Threshold_Time  SampleTime=-1  mask(TL_Constant){data={'output',{'variable','DEMO_FAS/p/Components/DEMO_FAS_Accusti_Threshold_Time'},'date',735382.58424127311}}
      | Constant block of dSPACE TargetLink.
      | 
      | Output signal keeps the given constant value.
      settings: DeleteFcn=if exist('delete_tlblock','file')==2,delete_tlblock(gcbh);end  NameChangeFcn=if exist('rename_tlblock','file')==2,rename_tlblock(gcbh);end  OpenFcn=if exist('tl_open_blockdlg','file')==2,tl_open_blockdlg(gcbh);else,open_system(gcbh,'parameter');end
      mask Help: eval(['if exist(''tl_online_help'',''file'') == 2, tl_online_help(''Topic'',''TL_Constant''),else, web([''jar:file:///'',matlabroot,''/help/toolbox/simulink/help.jar!/slref/' lower(get_param(gcbh,'Blocktype')) '.html''], ''-helpbrowser''),end'])
      mask Display: plot([-0.05, 1.05, NaN, -0.05, 1.05],[.01, .01, NaN, .99, .99])
  DEMO_FAS_Opti_Threshold_Time : Constant  Description=|  Value=DEMO_FAS_Opti_Threshold_Time  SampleTime=-1  mask(TL_Constant){data={'output',{'variable','DEMO_FAS/p/Components/DEMO_FAS_Opti_Threshold_Time'},'date',735382.58416377311}}
      | Constant block of dSPACE TargetLink.
      | 
      | Output signal keeps the given constant value.
      settings: DeleteFcn=if exist('delete_tlblock','file')==2,delete_tlblock(gcbh);end  NameChangeFcn=if exist('rename_tlblock','file')==2,rename_tlblock(gcbh);end  OpenFcn=if exist('tl_open_blockdlg','file')==2,tl_open_blockdlg(gcbh);else,open_system(gcbh,'parameter');end
      mask Help: eval(['if exist(''tl_online_help'',''file'') == 2, tl_online_help(''Topic'',''TL_Constant''),else, web([''jar:file:///'',matlabroot,''/help/toolbox/simulink/help.jar!/slref/' lower(get_param(gcbh,'Blocktype')) '.html''], ''-helpbrowser''),end'])
      mask Display: plot([-0.05, 1.05, NaN, -0.05, 1.05],[.01, .01, NaN, .99, .99])
  Mul : Product  Description=|  Inputs=**  RndMeth=Zero  mask(TL_Product){data={'logdata',{'plotchannels',[]},'date',734383.73388434027}}
      | Product block of dSPACE TargetLink.
      | 
      | Output signal is equal to the product of the input signals. The input ports are specified according to conventions for Simulink Product blocks.
      settings: CopyFcn=if exist('tl_reset_reviewflag') == 2, tl_reset_reviewflag(gcbh); end  DeleteFcn=if exist('delete_tlblock','file')==2,delete_tlblock(gcbh);end  NameChangeFcn=if exist('rename_tlblock','file')==2,rename_tlblock(gcbh);end  OpenFcn=if exist('tl_open_blockdlg','file')==2,tl_open_blockdlg(gcbh);else,open_system(gcbh,'parameter');end
      mask Help: eval(['if exist(''tl_online_help'',''file'') == 2, tl_online_help(''Topic'',''TL_Product''),else, web([''jar:file:///'',matlabroot,''/help/toolbox/simulink/help.jar!/slref/' lower(get_param(gcbh,'Blocktype')) '.html''], ''-helpbrowser''),end'])
      mask Display: plot([-0.05, 1.05, NaN, -0.05, 1.05],[.01, .01, NaN, .99, .99])
  Mul1 : Product  Description=|  Inputs=**  RndMeth=Zero  mask(TL_Product){data={'logdata',{'plotchannels',[]},'date',734383.73388434027}}
      | Product block of dSPACE TargetLink.
      | 
      | Output signal is equal to the product of the input signals. The input ports are specified according to conventions for Simulink Product blocks.
      settings: CopyFcn=if exist('tl_reset_reviewflag') == 2, tl_reset_reviewflag(gcbh); end  DeleteFcn=if exist('delete_tlblock','file')==2,delete_tlblock(gcbh);end  NameChangeFcn=if exist('rename_tlblock','file')==2,rename_tlblock(gcbh);end  OpenFcn=if exist('tl_open_blockdlg','file')==2,tl_open_blockdlg(gcbh);else,open_system(gcbh,'parameter');end
      mask Help: eval(['if exist(''tl_online_help'',''file'') == 2, tl_online_help(''Topic'',''TL_Product''),else, web([''jar:file:///'',matlabroot,''/help/toolbox/simulink/help.jar!/slref/' lower(get_param(gcbh,'Blocktype')) '.html''], ''-helpbrowser''),end'])
      mask Display: plot([-0.05, 1.05, NaN, -0.05, 1.05],[.01, .01, NaN, .99, .99])
  RelOp : RelationalOperator  Description=|  Operator=<=  mask(TL_RelationalOperator){data={'logdata',{'plotchannels',[]},'date',734383.73388379626}}
      | Relational operator block of dSPACE TargetLink.
      | 
      | This block performs a relational operation on its two inputs u1 and u2 and produces output according to the following table.
      | If the result is TRUE, the output is 1; if FALSE, it is 0.
      | 
      | Operator   Output
      |  ==        TRUE if u1 is equal to u2
      |  !=        TRUE if u1 is not equal to u2
      |  <         TRUE if u1 is less than u2
      |  <=        TRUE if u1 is less than or equal to u2
      |  >=        TRUE if u1 is greater than or equal to u2
      |  >         TRUE if u1 is greater than u2
      settings: DeleteFcn=if exist('delete_tlblock','file')==2,delete_tlblock(gcbh);end  NameChangeFcn=if exist('rename_tlblock','file')==2,rename_tlblock(gcbh);end  OpenFcn=if exist('tl_open_blockdlg','file')==2,tl_open_blockdlg(gcbh);else,open_system(gcbh,'parameter');end
      mask Help: eval(['if exist(''tl_online_help'',''file'') == 2, tl_online_help(''Topic'',''TL_RelationalOperator''),else, web([''jar:file:///'',matlabroot,''/help/toolbox/simulink/help.jar!/slref/' lower(get_param(gcbh,'Blocktype')) '.html''], ''-helpbrowser''),end'])
      mask Display: plot([-0.05, 1.05, NaN, -0.05, 1.05],[.01, .01, NaN, .99, .99])
  RelOp2 : RelationalOperator  Description=|  Operator=<=  mask(TL_RelationalOperator){data={'logdata',{'plotchannels',[]},'date',734383.73388379626}}
      | Relational operator block of dSPACE TargetLink.
      | 
      | This block performs a relational operation on its two inputs u1 and u2 and produces output according to the following table.
      | If the result is TRUE, the output is 1; if FALSE, it is 0.
      | 
      | Operator   Output
      |  ==        TRUE if u1 is equal to u2
      |  !=        TRUE if u1 is not equal to u2
      |  <         TRUE if u1 is less than u2
      |  <=        TRUE if u1 is less than or equal to u2
      |  >=        TRUE if u1 is greater than or equal to u2
      |  >         TRUE if u1 is greater than u2
      settings: DeleteFcn=if exist('delete_tlblock','file')==2,delete_tlblock(gcbh);end  NameChangeFcn=if exist('rename_tlblock','file')==2,rename_tlblock(gcbh);end  OpenFcn=if exist('tl_open_blockdlg','file')==2,tl_open_blockdlg(gcbh);else,open_system(gcbh,'parameter');end
      mask Help: eval(['if exist(''tl_online_help'',''file'') == 2, tl_online_help(''Topic'',''TL_RelationalOperator''),else, web([''jar:file:///'',matlabroot,''/help/toolbox/simulink/help.jar!/slref/' lower(get_param(gcbh,'Blocktype')) '.html''], ''-helpbrowser''),end'])
      mask Display: plot([-0.05, 1.05, NaN, -0.05, 1.05],[.01, .01, NaN, .99, .99])
  VERSION_INFO : Subsystem  mask(VERSION_INFO_BLOCK){versinfo_data=struct('modname','DEMO_FAS/DEMO_FAS_Funktion/Distancewarner/Distancewarner_Function','version','1.1.1','date','23-May-2013','author','YVEDUHR','modtype',3,'variant',0,'remark',{{'~'}},'copyright',['Daimler AG'],'SGMLdescr','','prefix','','pfx_act',0,'ntselect',3,'asize',0), versinfo_string=Model: DEMO_FAS/DEMO_FAS_Funktion/Distancewarner/Distancewarner_Function\nVersion: 1.1.1\nDate: 23-May-2013\nAuthor: YVEDUHR\nModule: INTERNAL\n\nAll copyrights by Daimler AG}
      mask prompts: versinfo_data "Mask Parameter 1"; versinfo_string "Mask Parameter 2"
      mask help:
      | This is a Version Info Subsystem (empty)
      | All version Information is stored in Parameter "versinfo_data" and displayed
      settings: OpenFcn=edit_subsys_info('init')
      mask Display: disp(versinfo_string);
  Opti_warn_b : Outport  OutputWhenDisabled=reset  InitialOutput=0
  Acusti_warn_b : Outport  Port=2  OutputWhenDisabled=reset  InitialOutput=0
  wires:
  V_Vehicle_ms/1 -> Mul/1, Mul1/1
  DEMO_FAS_Opti_Threshold_Time/1 -> Mul/2
  RelOp/1 -> Opti_warn_b/1  "Opti_warn_b"
  Mul/1 -> RelOp/2  "opti_warn_b"
  Distance_Object_m/1 -> RelOp2/1, RelOp/1
  RelOp2/1 -> Acusti_warn_b/1  "Acusti_warn_b"
  DEMO_FAS_Accusti_Threshold_Time/1 -> Mul1/2
  Mul1/1 -> RelOp2/2

== system DAS/DEMO_FAS/DEMO_FAS/Subsystem/DEMO_FAS/DEMO_FAS_Funktion/Distancewarner/VERSION_INFO ==
  Copyright : Subsystem
      mask help: Copyright
      mask Display: disp('All copyrights by DaimlerChrysler');
